simulink model "W01_Base_World_real_time_low_res_cs"  (R2019a)
settings: Solver=FixedStepDiscrete  StartTime=0.0  StopTime=100  FixedStep=1/10  RelTol=1e-3
PreLoadFcn:
  | mbxruntime.callbacks.PreLoadFcn(bdroot);
  | check_NUTS_defined
  | model_closed = 0;
  | assignin('base',['model_closed_' bdroot],false);
PostLoadFcn:
  | mbxruntime.callbacks.PostLoadFcn(bdroot);
InitFcn:
  | mbxruntime.callbacks.InitFcn(bdroot);
StartFcn:
  | mbxruntime.callbacks.StartFcn(bdroot);
StopFcn:
  | mbxruntime.callbacks.StopFcn(bdroot);;
  | 
model workspace: external: MAT-File .\W01_Base_World_real_time_low_res_cs_hws.mat (data not in the file)
undefined symbols (not defined in the file): DiscIntNeverNeededParam, Header, InitImageOutputDir, mbxruntime, Orientation, Poses, Poses_SL_Info, Position, tabledata, W01_Base_World_real_time_low_res_cs_07839109b96a80ba, W01_Base_World_real_time_low_res_cs_0c43d3473a460476, W01_Base_World_real_time_low_res_cs_0cf86600f728d0b5, W01_Base_World_real_time_low_res_cs_177a09ed8ce5b926, W01_Base_World_real_time_low_res_cs_220c936d9a28d27f, W01_Base_World_real_time_low_res_cs_2baf91e46e7f2a04, W01_Base_World_real_time_low_res_cs_3233ee773087b125, W01_Base_World_real_time_low_res_cs_3b004e0a9768fcfb, W01_Base_World_real_time_low_res_cs_3c5b4c2e4fe1a239, W01_Base_World_real_time_low_res_cs_3f14acb16f4df02a, W01_Base_World_real_time_low_res_cs_41ea08bfb3df5e8e, W01_Base_World_real_time_low_res_cs_5b313be3db799010, W01_Base_World_real_time_low_res_cs_6023c8b3cbf5a6a9, W01_Base_World_real_time_low_res_cs_6e743a938f29deb3, W01_Base_World_real_time_low_res_cs_8fce487235efddd0, W01_Base_World_real_time_low_res_cs_9d035aa0b54c0e3f, W01_Base_World_real_time_low_res_cs_d2428e0262163214, W01_Base_World_real_time_low_res_cs_d6d3920523b4384a, W01_Base_World_real_time_low_res_cs_fd401d13d3341c0a, W01_Base_World_real_time_low_res_cs_fe3582372ea2aab5
libraries: adeye_lib x37, simulink_extras x30, simulink x10, robotlib x4, sharedtransform x2, PreScanSimulinkLibrary x2
(part 2 of 8)

== system W01_Base_World_real_time_low_res_cs/ANIM_Child_RegularAni_1 ==
  ANIM_Child_RegularAni_1 : Inport  Tag=inport/AnimationOutport  OutDataTypeStr=Bus: PRESCAN_ANIMACTUATORDATA  PortDimensions=1  SampleTime=1/10  BusOutputAsStruct=on
  Actuator : S-Function  FunctionName=sfun_AnimActuator  Parameters=mbxruntime.parameters.convert(UniqueID), mbxruntime.parameters.convert(TimeStep)  SFunctionDeploymentMode=off  EnableBusSupport=off  mask(PreScan Sink Block: State Animation){UniqueID=18395, TimeStep=1/10}
      mask prompts: UniqueID "Auto-Assigned: Unique ID"; TimeStep "Auto-Assigned: Upload Period [s]"
      mask help: The Human Animation port allows the human to walk, run or bend
      mask Help: eval('openHelp(239)')
      mask Display: image(imread('HumanAnimated.jpg'))
  wires:
  ANIM_Child_RegularAni_1/1 -> Actuator/1

== system W01_Base_World_real_time_low_res_cs/ANIM_Child_RegularAni_2 ==
  ANIM_Child_RegularAni_2 : Inport  Tag=inport/AnimationOutport  OutDataTypeStr=Bus: PRESCAN_ANIMACTUATORDATA  PortDimensions=1  SampleTime=1/10  BusOutputAsStruct=on
  Actuator : S-Function  FunctionName=sfun_AnimActuator  Parameters=mbxruntime.parameters.convert(UniqueID), mbxruntime.parameters.convert(TimeStep)  SFunctionDeploymentMode=off  EnableBusSupport=off  mask(PreScan Sink Block: State Animation){UniqueID=18628, TimeStep=1/10}
      mask prompts: UniqueID "Auto-Assigned: Unique ID"; TimeStep "Auto-Assigned: Upload Period [s]"
      mask help: The Human Animation port allows the human to walk, run or bend
      mask Help: eval('openHelp(239)')
      mask Display: image(imread('HumanAnimated.jpg'))
  wires:
  ANIM_Child_RegularAni_2/1 -> Actuator/1

== system W01_Base_World_real_time_low_res_cs/ANIM_Female_RegularAni_1 ==
  ANIM_Female_RegularAni_1 : Inport  Tag=inport/AnimationOutport  OutDataTypeStr=Bus: PRESCAN_ANIMACTUATORDATA  PortDimensions=1  SampleTime=1/10  BusOutputAsStruct=on
  Actuator : S-Function  FunctionName=sfun_AnimActuator  Parameters=mbxruntime.parameters.convert(UniqueID), mbxruntime.parameters.convert(TimeStep)  SFunctionDeploymentMode=off  EnableBusSupport=off  mask(PreScan Sink Block: State Animation){UniqueID=18631, TimeStep=1/10}
      mask prompts: UniqueID "Auto-Assigned: Unique ID"; TimeStep "Auto-Assigned: Upload Period [s]"
      mask help: The Human Animation port allows the human to walk, run or bend
      mask Help: eval('openHelp(239)')
      mask Display: image(imread('HumanAnimated.jpg'))
  wires:
  ANIM_Female_RegularAni_1/1 -> Actuator/1

== system W01_Base_World_real_time_low_res_cs/ANIM_Male_RegularAni_1 ==
  ANIM_Male_RegularAni_1 : Inport  Tag=inport/AnimationOutport  OutDataTypeStr=Bus: PRESCAN_ANIMACTUATORDATA  PortDimensions=1  SampleTime=1/10  BusOutputAsStruct=on
  Actuator : S-Function  FunctionName=sfun_AnimActuator  Parameters=mbxruntime.parameters.convert(UniqueID), mbxruntime.parameters.convert(TimeStep)  SFunctionDeploymentMode=off  EnableBusSupport=off  mask(PreScan Sink Block: State Animation){UniqueID=18634, TimeStep=1/10}
      mask prompts: UniqueID "Auto-Assigned: Unique ID"; TimeStep "Auto-Assigned: Upload Period [s]"
      mask help: The Human Animation port allows the human to walk, run or bend
      mask Help: eval('openHelp(239)')
      mask Display: image(imread('HumanAnimated.jpg'))
  wires:
  ANIM_Male_RegularAni_1/1 -> Actuator/1

== system W01_Base_World_real_time_low_res_cs/ANIM_Male_RegularAni_2 ==
  ANIM_Male_RegularAni_2 : Inport  Tag=inport/AnimationOutport  OutDataTypeStr=Bus: PRESCAN_ANIMACTUATORDATA  PortDimensions=1  SampleTime=1/10  BusOutputAsStruct=on
  Actuator : S-Function  FunctionName=sfun_AnimActuator  Parameters=mbxruntime.parameters.convert(UniqueID), mbxruntime.parameters.convert(TimeStep)  SFunctionDeploymentMode=off  EnableBusSupport=off  mask(PreScan Sink Block: State Animation){UniqueID=18853, TimeStep=1/10}
      mask prompts: UniqueID "Auto-Assigned: Unique ID"; TimeStep "Auto-Assigned: Upload Period [s]"
      mask help: The Human Animation port allows the human to walk, run or bend
      mask Help: eval('openHelp(239)')
      mask Display: image(imread('HumanAnimated.jpg'))
  wires:
  ANIM_Male_RegularAni_2/1 -> Actuator/1

== system W01_Base_World_real_time_low_res_cs/Audi_A8_Sedan_1 ==
  SELF_Audi_A8_Sedan_1 : Inport  Tag=inport/SelfPort  OutDataTypeStr=Bus: PRESCAN_SELFSENSORDATA  PortDimensions=1  SampleTime=1/10  BusOutputAsStruct=on
  Car_Pos_and_Orient : Subsystem
  Path : S-Function  LoadFcn=load('PrescanMotionData.mat')  FunctionName=sfun_Path  Parameters=mbxruntime.parameters.convert(uniqueID), pathUniqueID, mbxruntime.parameters.convert(timestep)  SFunctionDeploymentMode=off  EnableBusSupport=off  mask(Path){uniqueID=18645, pathUniqueID=W01_Base_World_real_time_low_res_cs_6e743a938f29deb3, timestep=1/10}
      mask prompts: uniqueID "Object Unique ID"; pathUniqueID "Path Unique ID"; timestep "MATLAB timestep:"
      mask help:
      | The path block outputs the position along a given trajectory.
      |
      | For more information, please click Help.
      mask Help: eval('openHelp(312)')
      mask Display: image(imread('Path.png'))
  SELF_Demux : Subsystem  Tag=demux/SelfPort  mask(PreScan Demux Block:){}
      mask help:
      | The SELF port shows (state) information of the actor itself. The outputs are position in the experiment's axis system and the GPS coordinates, and the object's absolute velocity and compass heading.
      |
      | For more information, please click Help.
      settings: DeleteFcn=PreScanBlockDeleteFcn;
      mask Help: eval('openHelp(462)')
      mask Display:
      | port_label('output',1,'x [m]')
      | port_label('output',2,'y [m]')
      | port_label('output',3,'z [m]','texmode','on')
      | port_label('output',4,'Rotx [deg]','texmode','on')
      | port_label('output',5,'Roty [deg]','texmode','on')
      | port_label('output',6,'Rotz [deg]','texmode','on')
      | port_label('output',7,'GPS lat [deg]','texmode','on')
      | port_label('output',8,'GPS long [deg]','texmode','on')
      | port_label('output',9,'GPS alt [m]','texmode','on')
      | port_label('output',10,'Velocity [m/s]')
      | port_label('output',11,'Heading [deg]')
      | port_label('output',12,'Yaw rate [deg/s]')
      | port_label('output',13,'Timestamp [s]')
  STATE_Audi_A8_Sedan_1_rc : RateTransition  Tag=mux_rc/StatePort  OutPortSampleTimeOpt=Inherit
  SpeedProfile : S-Function  LoadFcn=load('PrescanMotionData.mat')  FunctionName=sfun_SpeedProfile  Parameters=speedProfileUniqueID, mbxruntime.parameters.convert(timestep)  SFunctionDeploymentMode=off  EnableBusSupport=off  mask(SpeedProfile){speedProfileUniqueID=W01_Base_World_real_time_low_res_cs_2baf91e46e7f2a04, timestep=1/10}
      mask prompts: speedProfileUniqueID "Speed Profile Unique ID"; timestep "MATLAB timestep:"
      mask help:
      | The speed profile block outputs the travelled distance, velocities and acceleration along a given path.
      |
      | For more information, please click Help.
      mask Help: eval('openHelp(312)')
      mask Display: image(imread('SpeedProfile.png'))
  Terminator_{1..7} (7 alike) : Terminator
  message_creator : Subsystem
  STATE_Audi_A8_Sedan_1_bus : Outport  Tag=outport/StatePort  OutDataTypeStr=Bus: PRESCAN_STATEACTUATORDATA  PortDimensions=1  SampleTime=1/10
  SafetyPlannerLoc : Outport  Port=2
  wires:
  Car_Pos_and_Orient/1(Out1) -> message_creator/1(In1)
  message_creator/1(Out1) -> SafetyPlannerLoc/1
  SELF_Demux/1(x [m]) -> Car_Pos_and_Orient/1(In1)
  SELF_Demux/2(y [m]) -> Car_Pos_and_Orient/2(In2)
  SELF_Demux/3(z [m]) -> Car_Pos_and_Orient/3(In3)
  SELF_Demux/4(rotx [deg]) -> Car_Pos_and_Orient/4(In4)
  SELF_Demux/5(roty [deg]) -> Car_Pos_and_Orient/5(In5)
  SELF_Demux/6(rotz [deg]) -> Car_Pos_and_Orient/6(In6)
  STATE_Audi_A8_Sedan_1_rc/1 -> STATE_Audi_A8_Sedan_1_bus/1
  SpeedProfile/1 -> Path/1
  Path/1 -> STATE_Audi_A8_Sedan_1_rc/1
  SELF_Audi_A8_Sedan_1/1 -> SELF_Demux/1(SELF)
  SELF_Demux/7(GPS lat [deg]) -> Terminator_1/1
  SELF_Demux/8(GPS long [deg]) -> Terminator_2/1
  SELF_Demux/9(GPS alt [m]) -> Terminator_3/1
  SELF_Demux/10(velocity [m/s]) -> Terminator_4/1
  SELF_Demux/11(heading [deg]) -> Terminator_5/1
  SELF_Demux/12(yaw rate [deg/s]) -> Terminator_6/1
  SELF_Demux/13(TimeStamp [s]) -> Terminator_7/1

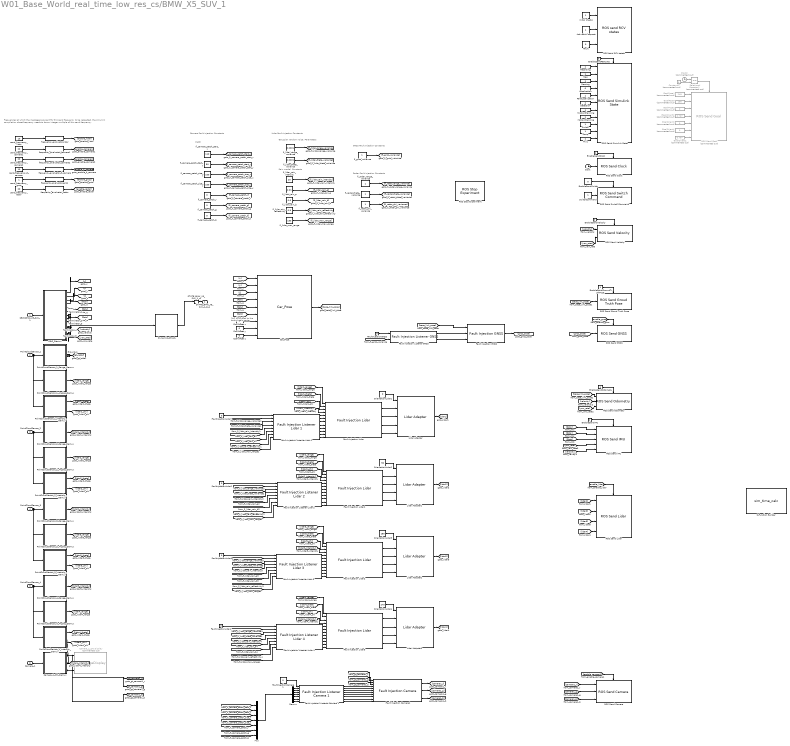
== system W01_Base_World_real_time_low_res_cs/BMW_X5_SUV_1 ==
  note: Frequencies at which the messages are sent
      |
      | For this send frequency to be respected, the simulink compilation sheet frequency
      | needs to be an integer multiple of this send frequency.
  note: Lidar Fault injection Constants
  note: Camera Fault injection Constants
  note: Patch
  note: Rain model, Constants
  note: Radar Fault Injection Constants
  note: Gaussian random noise, Parameters
  note: GNSS Fault Injection Constants
  note: CoG  compared
      | to the backwheels
      | center
  SELF_BMW_X5_SUV_1 : Inport  Tag=inport/SelfPort  OutDataTypeStr=Bus: PRESCAN_SELFSENSORDATA  PortDimensions=1  SampleTime=1/10  BusOutputAsStruct=on
  PointCloudSensor_1 : Inport  Tag=inport/PointCloudInport  Port=2  OutDataTypeStr=single  SampleTime=1/10  BusOutputAsStruct=on
  PointCloudSensor_2 : Inport  Tag=inport/PointCloudInport  Port=3  OutDataTypeStr=single  SampleTime=1/10  BusOutputAsStruct=on
  PointCloudSensor_3 : Inport  Tag=inport/PointCloudInport  Port=4  OutDataTypeStr=single  SampleTime=1/10  BusOutputAsStruct=on
  PointCloudSensor_4 : Inport  Tag=inport/PointCloudInport  Port=5  OutDataTypeStr=single  SampleTime=1/10  BusOutputAsStruct=on
  Camera_1 : Inport  Tag=inport/Camera/CameraSensor  Port=6  OutDataTypeStr=uint8  SampleTime=1/10  BusOutputAsStruct=on
  Activation request : Constant  OutDataTypeStr=Inherit: Inherit via back propagation
  Camera_1_CM_Demux : Subsystem  Tag=demux/Camera/Color  mask{SensorName=Camera_1, hres=480, vres=360}
      mask prompts: SensorName "Sensor Name"; hres "Horizontal Resolution"; vres "Vertical Resolution"
      mask Help: eval('openHelp(457)')
      mask Display:
      | fprintf('MONO CAMERA:\n Color\n %s \n %d x %d px',SensorName,hres,vres)
      | port_label('output',1,'R')
      | port_label('output',2,'G')
      | port_label('output',3,'B')
  Camera_1_CM_Display : M-S-Function  Tag=CameraSensor_Color_Display  Commented=on  InitFcn=InitImageOutputDir(gcb);  FunctionName=fcn_ImageDisplay  Parameters=SensorName EnableDisplay EnablePosition DisplayPosition FigureHandle SaveResults BitmapFormat TempOutputDir CameraType DataType  mask(PreScan Color Display Block){SensorName=Camera_1, EnableDisplay=off, EnablePosition=off, DisplayPosition=[10 10 480 360], FigureHandle=904005, SaveResults=off, Format=PNG, TempOutputDir=0, CameraType=Mono, DataType=uint8}
      mask prompts: SensorName "User Specified: Title of Display"; EnableDisplay "Active"; EnablePosition "Set Display window position"; DisplayPosition "Display window position [xpos ypos width height]"; FigureHandle "Unique Handle"; SaveResults "Save results"; TempOutputDir "OutputDir"; CameraType "Camera Type"; DataType "Image Data Type"
      mask help: This block displays the RGB output of a PreScan camera sensor.
      mask init:
      | if EnableDisplay
      |     EnableString='';
      |     EnableColor='gray';
      | else
      |     EnableString='INACTIVE';
      |     EnableColor='red';
      | end
      | switch Format
      |     case 1
      |         BitmapFormat = 'png';
      |     case 2
      |         BitmapFormat = 'bmp';
      |     case 3
      |         BitmapFormat = 'jpg';
      | end 
      | if CameraType==1
      |     CameraTypeName='MONO';
      |     PortNumber=0;
      | else
      |     CameraTypeName='STEREO';
      |     PortNumber=3;
      | end
      settings: CopyFcn=CopyFcnDisplay  DeleteFcn=PreScanBlockDeleteFcn;  ModelCloseFcn=fcn_ImageDisplay_ModelCloseFcn
      mask Help: eval('openHelp(457)')
      mask Callback EnablePosition:
      | MV=get_param(gcb,'MaskVisibilities');
      | if strcmp(get_param(gcb,'EnablePosition'),'on')
      |     MV{4}='on';
      | else
      |     MV{4}='off';
      | end
      | set_param(gcb,'MaskVisibilities',MV);
      | clear MV;
      mask TypeOptions Format: PNG | BMP | JPG
      mask TypeOptions CameraType: Mono | Stereo
      mask TypeOptions DataType: uint8 | single
      mask Display:
      | color(EnableColor);
      | fprintf('%s\n DISPLAY:\n Color \n %s',EnableString,SensorName)
      | port_label('input',1,'R')
      | port_label('input',2,'G')
      | port_label('input',3,'B')
      | port_label('input',PortNumber+1,'R')
      | port_label('input',PortNumber+2,'G')
      | port_label('input',PortNumber+3,'B')
  Car_Pose : adeye_lib/Car_Pose  SystemSampleTime=-1
  Clock : Clock
  Clock2 : Clock  Commented=on
  CoG offset x : Constant  Value=0
  CoG offset y : Constant  Value=0
  CoG offset z : Constant  Value=0
  Constant27 : Constant  Commented=on  Value=0
  Demux : Demux  Outputs=7
  Detection : Constant
  Dynamics_Empty : Subsystem  Tag=Dynamics_Empty
      mask Help: eval('openHelp(202)')
      mask Display: port_label('output', 1, 'State');text(0,0,' Empty\n')
  EnableSendClock : Constant  OutDataTypeStr=Inherit: Inherit via back propagation
  EnableSendFeatures : Constant  Value=0  OutDataTypeStr=Inherit: Inherit via back propagation
  EnableSendGroundTruthPose : Constant
  EnableSendIMU : Constant  OutDataTypeStr=Inherit: Inherit via back propagation
  EnableSendOdometry : Constant
  EnableSendSwitch : Constant  Value=0  OutDataTypeStr=Inherit: Inherit via back propagation  SampleTime=-1
  EnableSendVelocity : Constant  OutDataTypeStr=Inherit: Inherit via back propagation
  FakeLocalization : Constant
  Fault : Constant  Value=0  OutDataTypeStr=Inherit: Inherit via back propagation
  Fault Injection Camera1 : adeye_lib/Fault Injection Camera  idy=200  idx=100  x=100  y=150  R=0  G=0  B=0
  Fault Injection GNSS : adeye_lib/Fault Injection GNSS  f=20
  Fault Injection Lidar{,1..3} (4 alike) : adeye_lib/Fault Injection Lidar  f=10  p=225*16
  Fault Injection Listener Camera 1 : adeye_lib/Fault Injection Listener Camera 1  SystemSampleTime=-1
  Fault Injection Listener GNSS : adeye_lib/Fault Injection Listener GNSS  SystemSampleTime=-1
  Fault Injection Listener Lidar 1 : adeye_lib/Fault Injection Listener Lidar 1  SystemSampleTime=-1
  Fault Injection Listener Lidar 2 : adeye_lib/Fault Injection Listener Lidar 2  SystemSampleTime=-1
  Fault Injection Listener Lidar 3 : adeye_lib/Fault Injection Listener Lidar 3  SystemSampleTime=-1
  Fault Injection Listener Lidar 4 : adeye_lib/Fault Injection Listener Lidar 4  SystemSampleTime=-1
  FaultInjectionCamera1 : Constant  Value=0
  FaultInjectionGNSS : Constant  Value=0  OutDataTypeStr=Inherit: Inherit via back propagation  SampleTime=-1
  FaultInjectionLidar{1..4} (4 alike) : Constant  Value=0  OutDataTypeStr=Inherit: Inherit via back propagation
  GoalOrientW : Constant  Commented=on  Value=0.707
  GoalOrientX : Constant  Commented=on  Value=0
  GoalOrientY : Constant  Commented=on  Value=0
  GoalOrientZ : Constant  Commented=on  Value=0.707
  GoalPoseX : Constant  Commented=on  Value=249
  GoalPoseY : Constant  Commented=on  Value=136
  GoalPoseZ : Constant  Commented=on  Value=0
  Ground_1 : Ground
  Initial checks : Constant  OutDataTypeStr=Inherit: Inherit via back propagation
  Lidar Adapter{,1..3} (4 alike) : adeye_lib/Lidar Adapter  SystemSampleTime=-1
  Localization : Constant  Value=0
  Map : Constant
  MissionPlanning : Constant
  MotionPlanning : Constant
  Mux : Mux  Inputs=7
  OrientationLidar1 : Constant  Value=0  OutDataTypeStr=Inherit: Inherit via back propagation
  OrientationLidar2 : Constant  Value=90  OutDataTypeStr=Inherit: Inherit via back propagation
  OrientationLidar3 : Constant  Value=180  OutDataTypeStr=Inherit: Inherit via back propagation
  OrientationLidar4 : Constant  Value=270  OutDataTypeStr=Inherit: Inherit via back propagation
  PointCloudSensor_1_Angles_Demux : Subsystem  Tag=demux/PCS/Angles  mask{SensorName=PointCloudSensor_1, offset=225, hres=225, vres=16}
      mask prompts: SensorName "Sensor Name"; offset "Data Start"; hres "Horizontal Resolution"; vres "Vertical Resolution"
      mask Help: eval('openHelp(6400)')
      mask Display:
      | fprintf('Point Cloud:\n Data\n %s \n %d x %d px',SensorName,hres,vres)
      | port_label('output',1,'Theta')
      | port_label('output',2,'Phi')
  PointCloudSensor_1_Intensity_Demux : Subsystem  Tag=demux/PCS/Intensity  mask{SensorName=PointCloudSensor_1, offset=675, hres=225, vres=16}
      mask prompts: SensorName "Sensor Name"; offset "Data Start"; hres "Horizontal Resolution"; vres "Vertical Resolution"
      mask Help: eval('openHelp(6400)')
      mask Display:
      | fprintf('Point Cloud:\n Data\n %s \n %d x %d px',SensorName,hres,vres)
      | port_label('output',1,'Intensity')
  PointCloudSensor_1_Range_Demux : Subsystem  Tag=demux/PCS/Range  mask{SensorName=PointCloudSensor_1, offset=0, hres=225, vres=16}
      mask prompts: SensorName "Sensor Name"; offset "Data Start"; hres "Horizontal Resolution"; vres "Vertical Resolution"
      mask Help: eval('openHelp(6400)')
      mask Display:
      | fprintf('Point Cloud:\n Data\n %s \n %d x %d px',SensorName,hres,vres)
      | port_label('output',1,'Range')
  PointCloudSensor_2_Angles_Demux : Subsystem  Tag=demux/PCS/Angles  mask{SensorName=PointCloudSensor_2, offset=225, hres=225, vres=16}
      mask prompts: SensorName "Sensor Name"; offset "Data Start"; hres "Horizontal Resolution"; vres "Vertical Resolution"
      mask Help: eval('openHelp(6400)')
      mask Display:
      | fprintf('Point Cloud:\n Data\n %s \n %d x %d px',SensorName,hres,vres)
      | port_label('output',1,'Theta')
      | port_label('output',2,'Phi')
  PointCloudSensor_2_Intensity_Demux : Subsystem  Tag=demux/PCS/Intensity  mask{SensorName=PointCloudSensor_2, offset=675, hres=225, vres=16}
      mask prompts: SensorName "Sensor Name"; offset "Data Start"; hres "Horizontal Resolution"; vres "Vertical Resolution"
      mask Help: eval('openHelp(6400)')
      mask Display:
      | fprintf('Point Cloud:\n Data\n %s \n %d x %d px',SensorName,hres,vres)
      | port_label('output',1,'Intensity')
  PointCloudSensor_2_Range_Demux : Subsystem  Tag=demux/PCS/Range  mask{SensorName=PointCloudSensor_2, offset=0, hres=225, vres=16}
      mask prompts: SensorName "Sensor Name"; offset "Data Start"; hres "Horizontal Resolution"; vres "Vertical Resolution"
      mask Help: eval('openHelp(6400)')
      mask Display:
      | fprintf('Point Cloud:\n Data\n %s \n %d x %d px',SensorName,hres,vres)
      | port_label('output',1,'Range')
  PointCloudSensor_3_Angles_Demux : Subsystem  Tag=demux/PCS/Angles  mask{SensorName=PointCloudSensor_3, offset=225, hres=225, vres=16}
      mask prompts: SensorName "Sensor Name"; offset "Data Start"; hres "Horizontal Resolution"; vres "Vertical Resolution"
      mask Help: eval('openHelp(6400)')
      mask Display:
      | fprintf('Point Cloud:\n Data\n %s \n %d x %d px',SensorName,hres,vres)
      | port_label('output',1,'Theta')
      | port_label('output',2,'Phi')
  PointCloudSensor_3_Intensity_Demux : Subsystem  Tag=demux/PCS/Intensity  mask{SensorName=PointCloudSensor_3, offset=675, hres=225, vres=16}
      mask prompts: SensorName "Sensor Name"; offset "Data Start"; hres "Horizontal Resolution"; vres "Vertical Resolution"
      mask Help: eval('openHelp(6400)')
      mask Display:
      | fprintf('Point Cloud:\n Data\n %s \n %d x %d px',SensorName,hres,vres)
      | port_label('output',1,'Intensity')
  PointCloudSensor_3_Range_Demux : Subsystem  Tag=demux/PCS/Range  mask{SensorName=PointCloudSensor_3, offset=0, hres=225, vres=16}
      mask prompts: SensorName "Sensor Name"; offset "Data Start"; hres "Horizontal Resolution"; vres "Vertical Resolution"
      mask Help: eval('openHelp(6400)')
      mask Display:
      | fprintf('Point Cloud:\n Data\n %s \n %d x %d px',SensorName,hres,vres)
      | port_label('output',1,'Range')
  PointCloudSensor_4_Angles_Demux : Subsystem  Tag=demux/PCS/Angles  mask{SensorName=PointCloudSensor_4, offset=225, hres=225, vres=16}
      mask prompts: SensorName "Sensor Name"; offset "Data Start"; hres "Horizontal Resolution"; vres "Vertical Resolution"
      mask Help: eval('openHelp(6400)')
      mask Display:
      | fprintf('Point Cloud:\n Data\n %s \n %d x %d px',SensorName,hres,vres)
      | port_label('output',1,'Theta')
      | port_label('output',2,'Phi')
  PointCloudSensor_4_Intensity_Demux : Subsystem  Tag=demux/PCS/Intensity  mask{SensorName=PointCloudSensor_4, offset=675, hres=225, vres=16}
      mask prompts: SensorName "Sensor Name"; offset "Data Start"; hres "Horizontal Resolution"; vres "Vertical Resolution"
      mask Help: eval('openHelp(6400)')
      mask Display:
      | fprintf('Point Cloud:\n Data\n %s \n %d x %d px',SensorName,hres,vres)
      | port_label('output',1,'Intensity')
  PointCloudSensor_4_Range_Demux : Subsystem  Tag=demux/PCS/Range  mask{SensorName=PointCloudSensor_4, offset=0, hres=225, vres=16}
      mask prompts: SensorName "Sensor Name"; offset "Data Start"; hres "Horizontal Resolution"; vres "Vertical Resolution"
      mask Help: eval('openHelp(6400)')
      mask Display:
      | fprintf('Point Cloud:\n Data\n %s \n %d x %d px',SensorName,hres,vres)
      | port_label('output',1,'Range')
  ROS Send Camera : adeye_lib/ROS Send Camera  SystemSampleTime=-1
  ROS Send Clock : adeye_lib/ROS Send Clock  Priority=1  SystemSampleTime=-1
  ROS Send GNSS : adeye_lib/ROS Send GNSS  SystemSampleTime=-1
  ROS Send Goal : adeye_lib/ROS Send Goal  Commented=on  SystemSampleTime=-1
  ROS Send Groud Truth Pose : adeye_lib/ROS Send Groud Truth Pose  SystemSampleTime=-1
  ROS Send IMU : adeye_lib/ROS Send IMU  SystemSampleTime=-1
  ROS Send Lidar : adeye_lib/ROS Send Lidar  SystemSampleTime=-1
  ROS Send Odometry : adeye_lib/ROS Send Odometry  SystemSampleTime=-1
  ROS Send Simulink State : adeye_lib/ROS Send Simulink State  SystemSampleTime=-1
  ROS Send Switch Command : adeye_lib/ROS Send Switch Command  SystemSampleTime=-1
  ROS Send Velocity : adeye_lib/ROS Send Velocity  SystemSampleTime=-1
  "ROS Stop Experiment " : adeye_lib/ROS Stop Experiment  SystemSampleTime=-1
  ROS send RCV states : adeye_lib/ROS send RCV states  SystemSampleTime=-1
  Recording : Constant
  Relational Operator1 : RelationalOperator  Commented=on  Operator===  OutDataTypeStr=boolean  RndMeth=Simplest
  Rviz : Constant
  S-Function Builder : S-Function  InitFcn=try, set_param(gcb,'FunctionName','sim_time_calc'), end  FunctionName=sim_time_calc  SFunctionModules=sim_time_calc_wrapper  SFunctionDeploymentMode=off  EnableBusSupport=off  mask(S-Function Builder){}
      mask help: Simulink:masks:SFunctionBuilder_MD
      mask init:
      | val = [[.9  0.75 0.75 1 1 .9 .9 1]',[1 1 0.75 0.75 .9 .9 1 .9]'];try , sys = get_param(gcb,'SfunBuilderFcnName');if isempty(sys), sys = get_param(gcb,'FunctionName'); end,catch, sys = get_param(gcb,'FunctionName'); end
      settings: CopyFcn=set_param(gcbh,'LinkStatus','none')  PreSaveFcn=try, set_param(gcb,'FunctionName','sim_time_calc'), end  OpenFcn=sfunctionwizard(gcbh)
      mask Display:
      | plot(val(:,1),val(:,2))
      | disp(sys)
  SELF_Demux : Subsystem  Tag=demux/SelfPort  mask(PreScan Demux Block:){}
      mask help:
      | The SELF port shows (state) information of the actor itself. The outputs are position in the experiment's axis system and the GPS coordinates, and the object's absolute velocity and compass heading.
      |
      | For more information, please click Help.
      settings: DeleteFcn=PreScanBlockDeleteFcn;
      mask Help: eval('openHelp(462)')
      mask Display:
      | port_label('output',1,'x [m]')
      | port_label('output',2,'y [m]')
      | port_label('output',3,'z [m]','texmode','on')
      | port_label('output',4,'Rotx [deg]','texmode','on')
      | port_label('output',5,'Roty [deg]','texmode','on')
      | port_label('output',6,'Rotz [deg]','texmode','on')
      | port_label('output',7,'GPS lat [deg]','texmode','on')
      | port_label('output',8,'GPS long [deg]','texmode','on')
      | port_label('output',9,'GPS alt [m]','texmode','on')
      | port_label('output',10,'Velocity [m/s]')
      | port_label('output',11,'Heading [deg]')
      | port_label('output',12,'Yaw rate [deg/s]')
      | port_label('output',13,'Timestamp [s]')
  STATE_BMW_X5_SUV_1_rc : RateTransition  Tag=mux_rc/StatePort  OutPortSampleTimeOpt=Inherit
  Sensing : Constant
  Ssmp : Constant
  Switch : Constant
  SwitchCommand : Constant  OutDataTypeStr=Inherit: Inherit via back propagation  SampleTime=-1
  Terminator_{1..5} (5 alike) : Terminator
  fi_camera_patch_b : Constant  Value=0
  fi_camera_patch_g : Constant  Value=0
  fi_camera_patch_r : Constant  Value=0
  fi_camera_patch_size_x : Constant  Value=100
  fi_camera_patch_size_y : Constant  Value=100
  fi_camera_patch_start_x : Constant  Value=110
  fi_camera_patch_start_y : Constant  Value=50
  fi_gnss_variance : Constant
  fi_lidar_max_range : Constant  Value=150
  fi_lidar_rain_a : Constant  Value=0.01
  fi_lidar_rain_b : Constant  Value=0.6
  fi_lidar_rain_intensity : Constant  Value=20
  fi_lidar_rain_reflectivity : Constant  Value=0.9
  fi_lidar_range_variance : Constant  Value=0.0001
  fi_lidar_theta_variance : Constant  Value=0.0001
  fi_radar_phi_variance : Constant
  fi_radar_range_variance : Constant
  fi_radar_theta_variance : Constant
  frequency_evaluator_camera1 : adeye_lib/frequency_evaluator  SystemSampleTime=-1
  frequency_evaluator_camera2 : adeye_lib/frequency_evaluator  SystemSampleTime=-1
  frequency_evaluator_gnss : adeye_lib/frequency_evaluator  SystemSampleTime=-1
  frequency_evaluator_lidar : adeye_lib/frequency_evaluator  SystemSampleTime=-1
      link override Constant: Value=0.999
  frequency_evaluator_radar : adeye_lib/frequency_evaluator  SystemSampleTime=-1
  frequency_evaluator_tl_camera : adeye_lib/frequency_evaluator  SystemSampleTime=-1
  send_frequency_camera1 : Constant  Priority=1  Value=20
  send_frequency_camera2 : Constant  Priority=1  Value=20
  send_frequency_gnss : Constant  Priority=1
  send_frequency_lidar : Constant  Priority=1  Value=10
  send_frequency_radar : Constant  Priority=1  Value=20
  send_frequency_tl_camera : Constant  Priority=1  Value=10
  STATE_BMW_X5_SUV_1_bus : Outport  Tag=outport/StatePort  OutDataTypeStr=Bus: PRESCAN_STATEACTUATORDATA  PortDimensions=1  SampleTime=1/10
  wires:
  Activation request/1 -> ROS send RCV states/2
  Initial checks/1 -> ROS send RCV states/1
  Fault/1 -> ROS send RCV states/3
  Car_Pose/1 -> [base_link_pose]
  [x] -> Car_Pose/1
  [y] -> Car_Pose/2
  [z] -> Car_Pose/3
  [Rotx] -> Car_Pose/4
  [Roty] -> Car_Pose/5
  [Rotz] -> Car_Pose/6
  CoG offset x/1 -> Car_Pose/7
  CoG offset y/1 -> Car_Pose/8
  CoG offset z/1 -> Car_Pose/9
  Clock/1 -> ROS Send Clock/1
  EnableSendClock/1 -> ROS Send Clock/Enable
  Clock2/1 -> Relational Operator1/1
  Relational Operator1/1 -> ROS Send Goal/Enable
  GoalPoseX/1 -> ROS Send Goal/1
  GoalPoseY/1 -> ROS Send Goal/2
  GoalPoseZ/1 -> ROS Send Goal/3
  GoalOrientW/1 -> ROS Send Goal/4
  GoalOrientX/1 -> ROS Send Goal/5
  GoalOrientY/1 -> ROS Send Goal/6
  GoalOrientZ/1 -> ROS Send Goal/7
  Constant27/1 -> Relational Operator1/2
  Demux/1 -> Fault Injection Listener Camera 1/2
  Fault Injection Listener Camera 1/1 -> Fault Injection Camera1/4
  Fault Injection Camera1/1 -> [camera1_r]
  Fault Injection Camera1/2 -> [camera1_g]
  Fault Injection Camera1/3 -> [camera1_b]
  [gt_camera1_r] -> Fault Injection Camera1/1
  [gt_camera1_g] -> Fault Injection Camera1/2
  [gt_camera1_b] -> Fault Injection Camera1/3
  Fault Injection Listener Camera 1/2 -> Fault Injection Camera1/5
  Fault Injection Listener Camera 1/3 -> Fault Injection Camera1/6
  Fault Injection Listener Camera 1/4 -> Fault Injection Camera1/7
  Fault Injection Listener Camera 1/5 -> Fault Injection Camera1/8
  Fault Injection Listener Camera 1/6 -> Fault Injection Camera1/9
  Fault Injection Listener Camera 1/7 -> Fault Injection Camera1/10
  Fault Injection Listener Camera 1/8 -> Fault Injection Camera1/11
  FaultInjectionCamera1/1 -> Fault Injection Listener Camera 1/1
  Demux/2 -> Fault Injection Listener Camera 1/3
  Demux/3 -> Fault Injection Listener Camera 1/4
  Demux/4 -> Fault Injection Listener Camera 1/5
  Demux/5 -> Fault Injection Listener Camera 1/6
  Demux/6 -> Fault Injection Listener Camera 1/7
  Demux/7 -> Fault Injection Listener Camera 1/8
  Mux/1 -> Demux/1
  [fi_camera_patch_start_x] -> Mux/1
  [fi_camera_patch_start_y] -> Mux/2
  [fi_camera_patch_size_x] -> Mux/3
  [fi_camera_patch_size_y] -> Mux/4
  [fi_camera_patch_r] -> Mux/5
  [fi_camera_patch_g] -> Mux/6
  [fi_camera_patch_b] -> Mux/7
  Detection/1 -> ROS Send Simulink State/6
  Recording/1 -> ROS Send Simulink State/1
  Map/1 -> ROS Send Simulink State/2
  Sensing/1 -> ROS Send Simulink State/3
  Localization/1 -> ROS Send Simulink State/4
  FakeLocalization/1 -> ROS Send Simulink State/5
  MissionPlanning/1 -> ROS Send Simulink State/7
  MotionPlanning/1 -> ROS Send Simulink State/8
  Switch/1 -> ROS Send Simulink State/9
  Ssmp/1 -> ROS Send Simulink State/10
  Rviz/1 -> ROS Send Simulink State/11
  EnableSendFeatures/1 -> ROS Send Simulink State/Enable
  [enable_camera1] -> ROS Send Camera/Enable
  [camera1_r] -> ROS Send Camera/1
  [camera1_g] -> ROS Send Camera/2
  [camera1_b] -> ROS Send Camera/3
  [enable_gnss] -> ROS Send GNSS/Enable
  [gnss_pose] -> ROS Send GNSS/1
  EnableSendIMU/1 -> ROS Send IMU/Enable
  [Rotx] -> ROS Send IMU/1
  [Roty] -> ROS Send IMU/2
  [Rotz] -> ROS Send IMU/3
  [yaw_rate] -> ROS Send IMU/4
  [velocity] -> ROS Send IMU/5
  [lidar1] -> ROS Send Lidar/1
  [lidar2] -> ROS Send Lidar/2
  [lidar3] -> ROS Send Lidar/3
  [lidar4] -> ROS Send Lidar/4
  EnableSendOdometry/1 -> ROS Send Odometry/Enable
  [base_link_pose] -> ROS Send Odometry/1
  [velocity] -> ROS Send Odometry/2
  [yaw_rate] -> ROS Send Odometry/3
  EnableSendSwitch/1 -> ROS Send Switch Command/Enable
  SwitchCommand/1 -> ROS Send Switch Command/1
  EnableSendVelocity/1 -> ROS Send Velocity/Enable
  [velocity] -> ROS Send Velocity/1
  [yaw_rate] -> ROS Send Velocity/2
  Fault Injection GNSS/1 -> [gnss_pose]
  [base_link_pose] -> Fault Injection GNSS/1
  Fault Injection Listener GNSS/1 -> Fault Injection GNSS/2
  Fault Injection Listener GNSS/2 -> Fault Injection GNSS/3
  FaultInjectionGNSS/1 -> Fault Injection Listener GNSS/1
  [fi_gnss_variance] -> Fault Injection Listener GNSS/2
  Fault Injection Lidar/1 -> Lidar Adapter/2
  Lidar Adapter/1 -> [lidar1]
  OrientationLidar1/1 -> Lidar Adapter/1
  Fault Injection Lidar/2 -> Lidar Adapter/3
  Fault Injection Lidar/3 -> Lidar Adapter/4
  Fault Injection Lidar/4 -> Lidar Adapter/5
  [lidar1_range] -> Fault Injection Lidar/1
  [lidar1_theta] -> Fault Injection Lidar/2
  [lidar1_phi] -> Fault Injection Lidar/3
  [lidar1_intensity] -> Fault Injection Lidar/4
  Fault Injection Listener Lidar 1/1 -> Fault Injection Lidar/5
  Fault Injection Listener Lidar 1/2 -> Fault Injection Lidar/6
  Fault Injection Listener Lidar 1/3 -> Fault Injection Lidar/7
  Fault Injection Listener Lidar 1/4 -> Fault Injection Lidar/8
  Fault Injection Listener Lidar 1/5 -> Fault Injection Lidar/9
  Fault Injection Listener Lidar 1/6 -> Fault Injection Lidar/10
  Fault Injection Listener Lidar 1/7 -> Fault Injection Lidar/11
  Fault Injection Listener Lidar 1/8 -> Fault Injection Lidar/12
  FaultInjectionLidar1/1 -> Fault Injection Listener Lidar 1/1
  [fi_lidar_range_variance] -> Fault Injection Listener Lidar 1/2
  [fi_lidar_theta_variance] -> Fault Injection Listener Lidar 1/3
  [fi_lidar_rain_intensity] -> Fault Injection Listener Lidar 1/4
  [fi_lidar_rain_a] -> Fault Injection Listener Lidar 1/5
  [fi_lidar_rain_b] -> Fault Injection Listener Lidar 1/6
  [fi_lidar_rain_reflectivity] -> Fault Injection Listener Lidar 1/7
  [fi_lidar_max_range] -> Fault Injection Listener Lidar 1/8
  Fault Injection Lidar1/1 -> Lidar Adapter1/2
  Lidar Adapter1/1 -> [lidar2]
  OrientationLidar2/1 -> Lidar Adapter1/1
  Fault Injection Lidar1/2 -> Lidar Adapter1/3
  Fault Injection Lidar1/3 -> Lidar Adapter1/4
  Fault Injection Lidar1/4 -> Lidar Adapter1/5
  [lidar2_range] -> Fault Injection Lidar1/1
  [lidar2_theta] -> Fault Injection Lidar1/2
  [lidar2_phi] -> Fault Injection Lidar1/3
  [lidar2_intensity] -> Fault Injection Lidar1/4
  Fault Injection Listener Lidar 2/1 -> Fault Injection Lidar1/5
  Fault Injection Listener Lidar 2/2 -> Fault Injection Lidar1/6
  Fault Injection Listener Lidar 2/3 -> Fault Injection Lidar1/7
  Fault Injection Listener Lidar 2/4 -> Fault Injection Lidar1/8
  Fault Injection Listener Lidar 2/5 -> Fault Injection Lidar1/9
  Fault Injection Listener Lidar 2/6 -> Fault Injection Lidar1/10
  Fault Injection Listener Lidar 2/7 -> Fault Injection Lidar1/11
  Fault Injection Listener Lidar 2/8 -> Fault Injection Lidar1/12
  FaultInjectionLidar2/1 -> Fault Injection Listener Lidar 2/1
  [fi_lidar_range_variance] -> Fault Injection Listener Lidar 2/2
  [fi_lidar_theta_variance] -> Fault Injection Listener Lidar 2/3
  [fi_lidar_rain_intensity] -> Fault Injection Listener Lidar 2/4
  [fi_lidar_rain_a] -> Fault Injection Listener Lidar 2/5
  [fi_lidar_rain_b] -> Fault Injection Listener Lidar 2/6
  [fi_lidar_rain_reflectivity] -> Fault Injection Listener Lidar 2/7
  [fi_lidar_max_range] -> Fault Injection Listener Lidar 2/8
  Fault Injection Lidar2/1 -> Lidar Adapter2/2
  Lidar Adapter2/1 -> [lidar3]
  OrientationLidar3/1 -> Lidar Adapter2/1
  Fault Injection Lidar2/2 -> Lidar Adapter2/3
  Fault Injection Lidar2/3 -> Lidar Adapter2/4
  Fault Injection Lidar2/4 -> Lidar Adapter2/5
  [lidar3_range] -> Fault Injection Lidar2/1
  [lidar3_theta] -> Fault Injection Lidar2/2
  [lidar3_phi] -> Fault Injection Lidar2/3
  [lidar3_intensity] -> Fault Injection Lidar2/4
  Fault Injection Listener Lidar 3/1 -> Fault Injection Lidar2/5
  Fault Injection Listener Lidar 3/2 -> Fault Injection Lidar2/6
  Fault Injection Listener Lidar 3/3 -> Fault Injection Lidar2/7
  Fault Injection Listener Lidar 3/4 -> Fault Injection Lidar2/8
  Fault Injection Listener Lidar 3/5 -> Fault Injection Lidar2/9
  Fault Injection Listener Lidar 3/6 -> Fault Injection Lidar2/10
  Fault Injection Listener Lidar 3/7 -> Fault Injection Lidar2/11
  Fault Injection Listener Lidar 3/8 -> Fault Injection Lidar2/12
  FaultInjectionLidar3/1 -> Fault Injection Listener Lidar 3/1
  [fi_lidar_range_variance] -> Fault Injection Listener Lidar 3/2
  [fi_lidar_theta_variance] -> Fault Injection Listener Lidar 3/3
  [fi_lidar_rain_intensity] -> Fault Injection Listener Lidar 3/4
  [fi_lidar_rain_a] -> Fault Injection Listener Lidar 3/5
  [fi_lidar_rain_b] -> Fault Injection Listener Lidar 3/6
  [fi_lidar_rain_reflectivity] -> Fault Injection Listener Lidar 3/7
  [fi_lidar_max_range] -> Fault Injection Listener Lidar 3/8
  Fault Injection Lidar3/1 -> Lidar Adapter3/2
  Lidar Adapter3/1 -> [lidar4]
  OrientationLidar4/1 -> Lidar Adapter3/1
  Fault Injection Lidar3/2 -> Lidar Adapter3/3
  Fault Injection Lidar3/3 -> Lidar Adapter3/4
  Fault Injection Lidar3/4 -> Lidar Adapter3/5
  [lidar4_range] -> Fault Injection Lidar3/1
  [lidar4_theta] -> Fault Injection Lidar3/2
  [lidar4_phi] -> Fault Injection Lidar3/3
  [lidar4_intensity] -> Fault Injection Lidar3/4
  Fault Injection Listener Lidar 4/1 -> Fault Injection Lidar3/5
  Fault Injection Listener Lidar 4/2 -> Fault Injection Lidar3/6
  Fault Injection Listener Lidar 4/3 -> Fault Injection Lidar3/7
  Fault Injection Listener Lidar 4/4 -> Fault Injection Lidar3/8
  Fault Injection Listener Lidar 4/5 -> Fault Injection Lidar3/9
  Fault Injection Listener Lidar 4/6 -> Fault Injection Lidar3/10
  Fault Injection Listener Lidar 4/7 -> Fault Injection Lidar3/11
  Fault Injection Listener Lidar 4/8 -> Fault Injection Lidar3/12
  FaultInjectionLidar4/1 -> Fault Injection Listener Lidar 4/1
  [fi_lidar_range_variance] -> Fault Injection Listener Lidar 4/2
  [fi_lidar_theta_variance] -> Fault Injection Listener Lidar 4/3
  [fi_lidar_rain_intensity] -> Fault Injection Listener Lidar 4/4
  [fi_lidar_rain_a] -> Fault Injection Listener Lidar 4/5
  [fi_lidar_rain_b] -> Fault Injection Listener Lidar 4/6
  [fi_lidar_rain_reflectivity] -> Fault Injection Listener Lidar 4/7
  [fi_lidar_max_range] -> Fault Injection Listener Lidar 4/8
  fi_camera_patch_b/1 -> [fi_camera_patch_b]
  fi_camera_patch_g/1 -> [fi_camera_patch_g]
  fi_camera_patch_r/1 -> [fi_camera_patch_r]
  fi_camera_patch_size_x/1 -> [fi_camera_patch_size_x]
  fi_camera_patch_size_y/1 -> [fi_camera_patch_size_y]
  fi_camera_patch_start_x/1 -> [fi_camera_patch_start_x]
  fi_camera_patch_start_y/1 -> [fi_camera_patch_start_y]
  fi_gnss_variance/1 -> [fi_gnss_variance]
  fi_lidar_max_range/1 -> [fi_lidar_max_range]
  fi_lidar_rain_a/1 -> [fi_lidar_rain_a]
  fi_lidar_rain_b/1 -> [fi_lidar_rain_b]
  fi_lidar_rain_intensity/1 -> [fi_lidar_rain_intensity]
  fi_lidar_rain_reflectivity/1 -> [fi_lidar_rain_reflectivity]
  fi_lidar_range_variance/1 -> [fi_lidar_range_variance]
  fi_lidar_theta_variance/1 -> [fi_lidar_theta_variance]
  fi_radar_phi_variance/1 -> [fi_radar_phi_variance]
  fi_radar_range_variance/1 -> [fi_radar_range_variance]
  fi_radar_theta_variance/1 -> [fi_radar_theta_variance]
  Camera_1_CM_Demux/3(B) -> [gt_camera1_b], Camera_1_CM_Display/3
  Camera_1_CM_Demux/2(G) -> [gt_camera1_g], Camera_1_CM_Display/2
  Camera_1_CM_Demux/1(R) -> [gt_camera1_r], Camera_1_CM_Display/1
  PointCloudSensor_1_Intensity_Demux/1(Intensity) -> [lidar1_intensity]
  PointCloudSensor_1_Angles_Demux/2(Phi) -> [lidar1_phi]
  PointCloudSensor_1_Range_Demux/1(Range) -> [lidar1_range]
  PointCloudSensor_1_Angles_Demux/1(Theta) -> [lidar1_theta]
  PointCloudSensor_2_Intensity_Demux/1(Intensity) -> [lidar2_intensity]
  PointCloudSensor_2_Angles_Demux/2(Phi) -> [lidar2_phi]
  PointCloudSensor_2_Range_Demux/1(Range) -> [lidar2_range]
  PointCloudSensor_2_Angles_Demux/1(Theta) -> [lidar2_theta]
  PointCloudSensor_3_Intensity_Demux/1(Intensity) -> [lidar3_intensity]
  PointCloudSensor_3_Angles_Demux/2(Phi) -> [lidar3_phi]
  PointCloudSensor_3_Range_Demux/1(Range) -> [lidar3_range]
  PointCloudSensor_3_Angles_Demux/1(Theta) -> [lidar3_theta]
  PointCloudSensor_4_Intensity_Demux/1(Intensity) -> [lidar4_intensity]
  PointCloudSensor_4_Angles_Demux/2(Phi) -> [lidar4_phi]
  PointCloudSensor_4_Range_Demux/1(Range) -> [lidar4_range]
  PointCloudSensor_4_Angles_Demux/1(Theta) -> [lidar4_theta]
  SELF_Demux/4(rotx [deg]) -> [Rotx]
  SELF_Demux/5(roty [deg]) -> [Roty]
  SELF_Demux/6(rotz [deg]) -> [Rotz]
  SELF_Demux/10(velocity [m/s]) -> [velocity], Dynamics_Empty/1(currant_speed)
  SELF_Demux/1(x [m]) -> [x]
  SELF_Demux/2(y [m]) -> [y]
  SELF_Demux/12(yaw rate [deg/s]) -> [yaw_rate]
  SELF_Demux/3(z [m]) -> [z]
  send_frequency_lidar/1 -> frequency_evaluator_lidar/1
  send_frequency_camera1/1 -> frequency_evaluator_camera1/1
  send_frequency_camera2/1 -> frequency_evaluator_camera2/1
  send_frequency_tl_camera/1 -> frequency_evaluator_tl_camera/1
  send_frequency_gnss/1 -> frequency_evaluator_gnss/1
  frequency_evaluator_lidar/1 -> [enable_lidar]
  frequency_evaluator_camera1/1 -> [enable_camera1]
  frequency_evaluator_camera2/1 -> [enable_camera2]
  frequency_evaluator_tl_camera/1 -> [enable_tl_camera]
  frequency_evaluator_gnss/1 -> [enable_gnss]
  [enable_lidar] -> ROS Send Lidar/Enable
  [base_link_pose] -> ROS Send Groud Truth Pose/1
  EnableSendGroundTruthPose/1 -> ROS Send Groud Truth Pose/Enable
  send_frequency_radar/1 -> frequency_evaluator_radar/1
  frequency_evaluator_radar/1 -> [enable_radar]
  STATE_BMW_X5_SUV_1_rc/1 -> STATE_BMW_X5_SUV_1_bus/1
  SELF_BMW_X5_SUV_1/1 -> SELF_Demux/1(SELF)
  PointCloudSensor_1/1 -> PointCloudSensor_1_Range_Demux/1(In1), PointCloudSensor_1_Angles_Demux/1(In2), PointCloudSensor_1_Intensity_Demux/1(In1)
  PointCloudSensor_2/1 -> PointCloudSensor_2_Range_Demux/1(In1), PointCloudSensor_2_Angles_Demux/1(In2), PointCloudSensor_2_Intensity_Demux/1(In1)
  PointCloudSensor_3/1 -> PointCloudSensor_3_Range_Demux/1(In1), PointCloudSensor_3_Angles_Demux/1(In2), PointCloudSensor_3_Intensity_Demux/1(In1)
  PointCloudSensor_4/1 -> PointCloudSensor_4_Range_Demux/1(In1), PointCloudSensor_4_Angles_Demux/1(In2), PointCloudSensor_4_Intensity_Demux/1(In1)
  Camera_1/1 -> Camera_1_CM_Demux/1(In1)
  Dynamics_Empty/1(State) -> STATE_BMW_X5_SUV_1_rc/1
  SELF_Demux/7(GPS lat [deg]) -> Terminator_1/1
  SELF_Demux/8(GPS long [deg]) -> Terminator_2/1
  SELF_Demux/9(GPS alt [m]) -> Terminator_3/1
  SELF_Demux/11(heading [deg]) -> Terminator_4/1
  SELF_Demux/13(TimeStamp [s]) -> Terminator_5/1
  Ground_1/1 -> [gt_radar]

== system W01_Base_World_real_time_low_res_cs/Camera_1 ==
  Sensor : S-Function  FunctionName=sfun_Camera  Parameters=mbxruntime.parameters.convert(sensorID), mbxruntime.parameters.convert(dataWidth), mbxruntime.parameters.convert(dataHeight), mbxruntime.parameters.convert(channelsPerImage), mbxruntime.parameters.convert(numberOfImages), mbxruntime.parameters.convert(timestep)  SFunctionDeploymentMode=off  EnableBusSupport=off  mask(PreScan Source Block: Camera Sensor){sensorID=9056, dataWidth=360, dataHeight=1440, channelsPerImage=3, numberOfImages=1, timestep=1/10}
      mask prompts: sensorID "Sensor ID"; dataWidth "Data width"; dataHeight "Data Height"; channelsPerImage "Channels per image"; numberOfImages "Number of images"; timestep "MATLAB timestep:"
      mask help: The Camera Sensor provides a color or monochrome image.
      mask Help: eval('openHelp(457)')
      mask Display: image(imread('CameraSensor.png'))
  Camera_1 : Outport  Tag=outport/Camera/CameraSensor  OutDataTypeStr=uint8  SampleTime=1/10
  wires:
  Sensor/1 -> Camera_1/1
